simulink model "DualSpin"  (R2019b)
settings: Solver=VariableStepAuto  StartTime=0.0  StopTime=10.0  RelTol=1e-3
values from neighbouring files (symbols this model uses):
  I_x = 0.07    [Lab_3.m]    (also in Lab_5.m)
  I_y = 0.0504    [Lab_3.m]    (also in Lab_5.m)
  I_z = 0.0109    [Lab_3.m]    (also in Lab_5.m)
undefined symbols (not defined in the file or in its folder): Ir
settings Model: Creator=adity  LastModifiedBy=adity

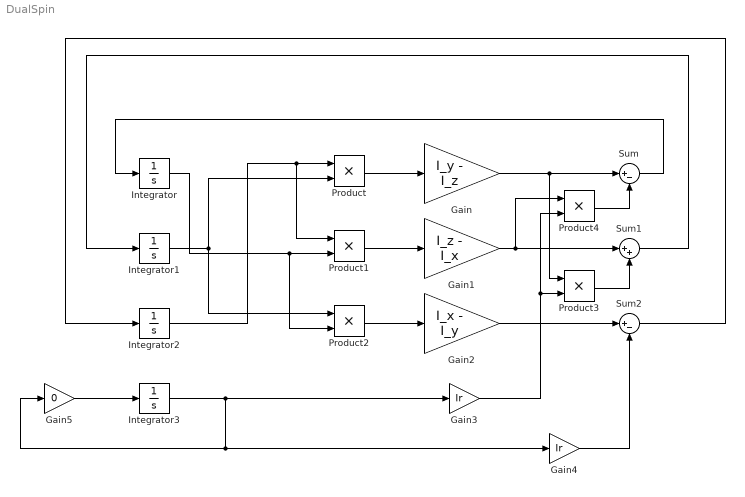
== system DualSpin ==
  Gain : Gain  Gain=I_y - I_z
  Gain1 : Gain  Gain=I_z - I_x
  Gain2 : Gain  Gain=I_x - I_y
  Gain3 : Gain  Gain=Ir
  Gain4 : Gain  Gain=Ir
  Gain5 : Gain  Gain=0
  Integrator{,1..3} (4 alike) : Integrator
  Product{,1..4} (5 alike) : Product
  Sum : Sum  Inputs=|+-
  Sum1 : Sum  Inputs=|++
  Sum2 : Sum  Inputs=|+-
  wires:
  Product/1 -> Gain/1
  Product1/1 -> Gain1/1
  Product2/1 -> Gain2/1
  Integrator2/1 -> Product1/1, Product/1
  Integrator1/1 -> Product2/1, Product/2
  Integrator/1 -> Product1/2, Product2/2
  Gain2/1 -> Sum2/1
  Gain1/1 -> Sum1/1, Product4/1
  Integrator3/1 -> Gain5/1, Gain4/1, Gain3/1
  Gain/1 -> Product3/1, Sum/1
  Gain4/1 -> Sum2/2
  Gain3/1 -> Product3/2, Product4/2
  Product4/1 -> Sum/2
  Product3/1 -> Sum1/2
  Sum/1 -> Integrator/1
  Sum1/1 -> Integrator1/1
  Sum2/1 -> Integrator2/1
  Gain5/1 -> Integrator3/1
